simulink model "case3"  (Simulink 5.0)
settings: Solver=ode15s  SolverMode=SingleTasking  StartTime=0.0  StopTime=2  RelTol=1e-4  AbsTol=1e-3
InitFcn:
  | powericon('psbinitsys',bdroot);
StopFcn:
  | set_param(gcs,'Dirty','off')
undefined symbols (not defined in the file): A11, A12, A13, A14, A15, A16, A21, A22, A23, A24, A25, A26, A31, A32, A33, A34, A35, A36, A41, A42, A43, A44, A45, A46, A51, A52, A53, A54, A55, A56, A61, A62, A63, A64, A65, A66, A67, A81, A82, A92, g1, g2, g4, g9, gref, Le, po, Re, u01, u02, Wr
libraries: powerlib2 x14
settings Model: RequirementInfo=9  Creator=patrice  LastModifiedBy=pavel  ExtModeTrigMode=oneshot  ExtModeArmWhenConnect=off  InitialState=xinit  SaveTime=off  SaveOutput=off  FinalStateName=xinit  LimitDataPoints=off  IntegerOverflowMsg=none  BlockReductionOpt=off  BooleanDataType=off  RTWTemplateMakefile=grt_unix.tmf

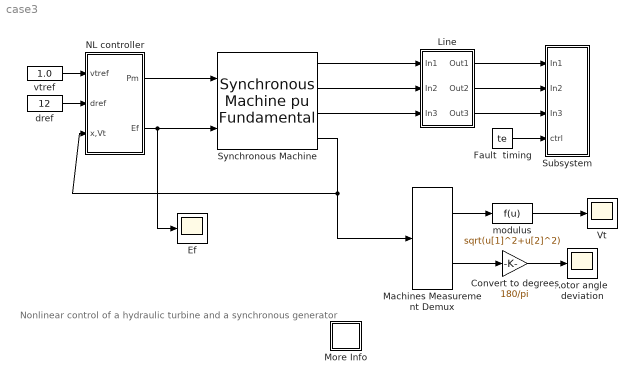
== system case3 ==
  note: Nonlinear control of a hydraulic turbine
      | and a synchronous generator
  Convert to degrees : Gain  Gain=180/pi  SaturateOnIntegerOverflow=on
  Ef : Scope
      settings: TickLabels=on  YMin=-12.5  YMax=12.5  DataFormat=Array
  Fault  timing : FromWorkspace  VariableName=te  SampleTime=0  mask( Fault timing){t=[0,0.1,0.2,0.4], e=[1,0,1,1]}
      mask prompts: t "transition steps:"; e "states (0/1):"
      mask help: steps
      mask init:
      | te=[t,t(2:length(t))-1e-8,t(length(t))+1e-8;e,e]';[y,i]=sort(te(:,1));te=[te(i,1),te(i,2)];
      mask Display: plot(te(:,1),te(:,2))
  Line : Subsystem
  Machines Measurement Demux : powerlib2/Machines/Machines Measurement Demux  machType=Synchronous  ssm1=on  ssm2=on  ssm3=on  ssm4=on  ssm5=on  ssm6=on  sm1=off  sm2=off  sm3=off  sm4=off  sm5=off  sm6=on  sm7=on  sm8=off  sm9=off  sm10=off  sm11=off  sm115=off  sm12=off  sm13=off  sm14=off  asm1=on  asm2=on  asm3=on  asm4=on  asm5=on  asm6=on  asm7=on  asm8=on  asm9=on  asm10=on  asm11=on  pmsm1=on  pmsm2=on  pmsm3=on  pmsm4=on  pmsm5=on  pmsm6=on  lastType=1
  More Info : Subsystem
      mask Display: disp('?')
  NL controller : Subsystem  mask(Non-linear speed and excitation controller){K=1, etat=1, mac=psbregulator/Synchronous Machine, delta=12, sm=[ 10/3  0.07 ], gate=[  0.01  0.97518  -0.1  0.1 ], Tw=2.67}
      mask prompts: K "Bus voltage (p.u.):"; etat "Controller state (0=off,1=on):"; mac "Associated machine name:"; delta "Desired load angle (deg):"; sm "Servo-motor [ Ka()  Ta(sec) ]:"; gate "Gate opening limits [ gmin,gmax(pu)    vgmin,vgmax(pu/s) ]:"; Tw "Water time constant Tw(sec):"
      mask init:
      | a=pi/2;[A11,A12,A13,A14,A15,A16,A21,A22,A23,A24,A25,A26,A31,A32,A33,A34,A35,A36,A41,A42,A43,A44,A45,A46,A51,A52,A53,A54,A55,A56,A61,A62,A63,A64,A65,A66,A67,A81,A82,A92,g1,g2,g4,g9,u01,u02,Re,Le,Wr,gref,po]=psbregulset(K,mac,delta);Ka=sm(1);Ta=sm(2);gmin=gate(1);gmax=gate(2);vgmin=gate(3);vgmax=gate(4);go=po*(gmax-gmin);
  Rotor angle  deviation : Scope
      settings: TickLabels=on  TimeRange=2  YMin=10.5  YMax=13.5  DataFormat=Array  Decimation=10
  Subsystem : Subsystem
  Synchronous Machine : powerlib2/Machines/Synchronous Machine pu Fundamental  Tag=PoWeRsYsTeMbLoCk  rotorType=Salient-pole  x1="[ 202E6  13800   60 ]"  x2="[ 0.003   0.19837   0.91763   0.21763 ]"  x3="[ 6.3581E-04   0.16537 ]"  x4b=[]  x4="[ 4.6454E-03  3.9203E-02  6.8430E-03  1.4544E-02 ]"  x5="[ 3.195  0  32 ]"  x6=[0 12 0.30512 0.30512 0.30512 105.77 -14.23 -134.23 0.970463]  x7=off  x8=[ ]  PSBOutputType=1110  iounits=0  LoadFlowParameters=[1,0,0,0,0]
  Vt : Scope
      settings: TickLabels=on  TimeRange=2  YMin=5.55112e-017  YMax=1.6  SaveName=ScopeData2  DataFormat=Array
  dref : Constant  Value=12
  modulus : Fcn  Expr=sqrt(u[1]^2+u[2]^2)
  vtref : Constant  Value=1.0
  wires:
  Synchronous Machine/3 -> Line/3(In3)
  Synchronous Machine/1 -> Line/1(In1)
  Synchronous Machine/2 -> Line/2(In2)
  Synchronous Machine/4 -> NL controller/3(x,Vt), Machines Measurement Demux/1
  dref/1 -> NL controller/2(dref)
  NL controller/2(Ef) -> Synchronous Machine/2, Ef/1
  vtref/1 -> NL controller/1(vtref)
  NL controller/1(Pm) -> Synchronous Machine/1
  Line/1(Out1) -> Subsystem/1(In1)
  Line/2(Out2) -> Subsystem/2(In2)
  Line/3(Out3) -> Subsystem/3(In3)
  Fault  timing/1 -> Subsystem/4(ctrl)
  Machines Measurement Demux/2 -> Convert to degrees/1
  Machines Measurement Demux/1 -> modulus/1
  modulus/1 -> Vt/1
  Convert to degrees/1 -> Rotor angle  deviation/1

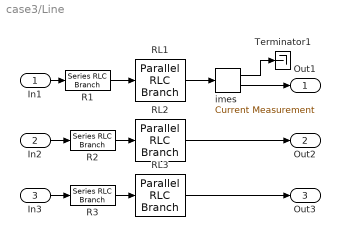
== system case3/Line ==
  In1 : Inport
  In2 : Inport  Port=2
  In3 : Inport  Port=3
  R1 : powerlib2/Elements/Series RLC Branch  Tag=PoWeRsYsTeMbLoCk  a=5.6566e-2  b=0  c=inf  mesure=None  PSBOutputType=1
  R2 : powerlib2/Elements/Series RLC Branch  Tag=PoWeRsYsTeMbLoCk  a=5.6566e-2  b=0  c=inf  mesure=None  PSBOutputType=1
  R3 : powerlib2/Elements/Series RLC Branch  Tag=PoWeRsYsTeMbLoCk  a=5.6566e-2  b=0  c=inf  mesure=None  PSBOutputType=1
  RL1 : powerlib2/Elements/Parallel RLC Branch  Tag=PoWeRsYsTeMbLoCk  a=25  b=6.5668e-4  c=0  mesure=None  PSBOutputType=1
  RL2 : powerlib2/Elements/Parallel RLC Branch  Tag=PoWeRsYsTeMbLoCk  a=25  b=6.5668e-4  c=0  mesure=None  PSBOutputType=1
  RL3 : powerlib2/Elements/Parallel RLC Branch  Tag=PoWeRsYsTeMbLoCk  a=25  b=6.5668e-4  c=0  mesure=None  PSBOutputType=1
  Terminator1 : Terminator
  imes : powerlib2/Measurements/Current Measurement  Tag=PoWeRsYsTeMmEaSuReMeNt  PhasorSimulation=off  OutputType=Magnitude  PSBOutputType=01  PSBequivalent=1
  Out1 : Outport  InitialOutput=0
  Out2 : Outport  Port=2  InitialOutput=0
  Out3 : Outport  Port=3  InitialOutput=0
  wires:
  imes/1 -> Terminator1/1
  RL3/1 -> Out3/1
  RL2/1 -> Out2/1
  In1/1 -> R1/1
  In2/1 -> R2/1
  In3/1 -> R3/1
  RL1/1 -> imes/1
  imes/2 -> Out1/1
  R1/1 -> RL1/1
  R2/1 -> RL2/1
  R3/1 -> RL3/1

== system case3/More Info ==
  note: Aime Francis Okou and Louis-A. Dessaint (École de technologie superieure, Montréal)
  note: 3
  note: Case study: Synchronous Machine and Regulator
  note: Circuit Description
  note: Demonstration
  note: This case study investigates the application of a multi-input multi-output nonlinear controller to a system consisting of a hydraulic
      | turbine and a synchronous generator connected to an infinite bus. The complete system is modeled using SimPowerSystems
      | and Simulink blocks. The controller is based on a feedback linearization scheme. Its main goal is to control the rotor angle as well as
      | the terminal voltage, to improve the stability properties, and to obtain good dynamic response.
      |
      | The performance of the nonlinear controller is tested on the nonlinear turbine-generator system. The controller and turbine are
      | simulated using Simulink blocks while the generator is represented by the Synchronous Machine block from the powerlib library.
      | A three-phase short-circuit is simulated on the load busbar and the fault is cleared after 100 ms.
  note: 1
  note: 2
  note: Start the simulation. Observe the field voltage Ef, power angle delta, and terminal voltage Vt.
  note: References
  note: You can observe how the stabilization of Vt is obtained in less than 0.25 seconds with this controller.
      | The load angle takes longer to stabilize, because the time constant of the mechanical part of the system
      | is much larger than the electrical time constants.
  note: If you want to compare results with classical regulators, replace the nonlinear controller with the same
      | excitation system and Hydraulic Turbine and Governor block used in the psbturbine demo. You will notice
      | that the system takes longer to stabilize than in this case study.
  note: Akhrif O., A.F. Okou, L.A. Dessaint, and R. Champagne, "Application of a Multivariable Feedback Linearization
      | Scheme for Rotor Angle Stability and Voltage Regulation of Power Systems", IEEE Transactions on Power Systems,
      | vol. 14, no. 2, May 1999, pp. 620-628.

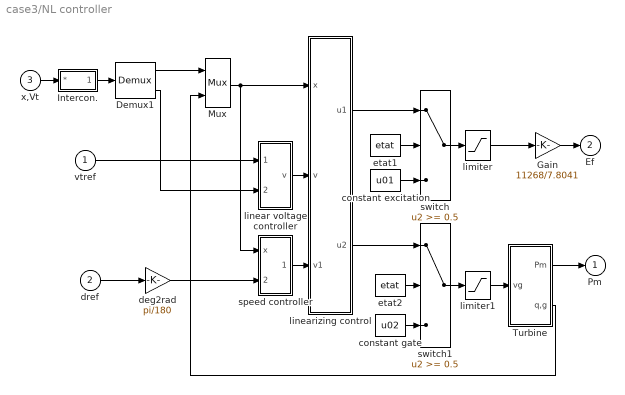
== system case3/NL controller ==
  vtref : Inport
  dref : Inport  Port=2
  x,Vt : Inport  Port=3
  Demux1 : Demux  Outputs=[7,1]
  Gain : Gain  Gain=11268/7.8041  SaturateOnIntegerOverflow=on
  Intercon. : Subsystem
  Mux : Mux  Inputs=[7,2]
  Turbine : Subsystem
  constant excitation : Constant  Value=u01
  constant gate : Constant  Value=u02
  deg2rad : Gain  Gain=pi/180  SaturateOnIntegerOverflow=on
  etat1 : Constant  Value=etat
  etat2 : Constant  Value=etat
  limiter : Saturate  UpperLimit=11.5*7.804/11268  LowerLimit=-11.5*7.804/11268  ZeroCross=off
  limiter1 : Saturate  UpperLimit=1  LowerLimit=-1  ZeroCross=off
  linear voltage controller : Subsystem
  linearizing control : Subsystem
  speed controller : Subsystem
  switch : Switch  Threshold=0.5  ZeroCross=off  InputSameDT=on
  switch1 : Switch  Threshold=0.5  ZeroCross=off  InputSameDT=on
  Pm : Outport  InitialOutput=0
  Ef : Outport  Port=2  InitialOutput=0
  wires:
  vtref/1 -> linear voltage controller/1(vtref)
  deg2rad/1 -> speed controller/2(dref)
  Gain/1 -> Ef/1
  Turbine/1(Pm) -> Pm/1
  constant gate/1 -> switch1/3
  etat2/1 -> switch1/2
  linearizing control/2(u2) -> switch1/1
  constant excitation/1 -> switch/3
  etat1/1 -> switch/2
  linearizing control/1(u1) -> switch/1
  switch1/1 -> limiter1/1
  limiter1/1 -> Turbine/1(vg)
  limiter/1 -> Gain/1
  switch/1 -> limiter/1
  linear voltage controller/1(v) -> linearizing control/2(v)
  speed controller/1(v1) -> linearizing control/3(v1)
  x,Vt/1 -> Intercon./1(*)
  Demux1/2 -> linear voltage controller/2(vt)
  Demux1/1 -> Mux/1
  Turbine/2(q,g) -> Mux/2
  dref/1 -> deg2rad/1
  Mux/1 -> linearizing control/1(x), speed controller/1(x)
  Intercon./1(" x,vt ") -> Demux1/1

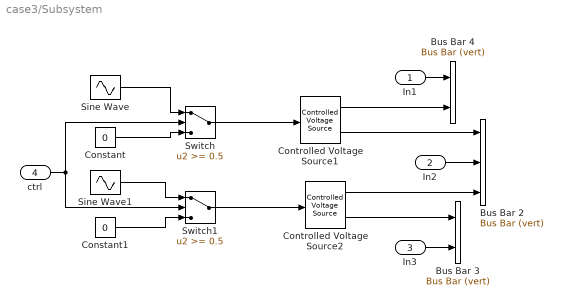
== system case3/Subsystem ==
  In1 : Inport
  In2 : Inport  Port=2
  In3 : Inport  Port=3
  ctrl : Inport  Port=4
  Bus Bar 2 : powerlib2/Connectors/Bus Bar (vert)  entrees=3  sorties=0  PSBOutputType=11111111111111111111111111111111111111111111111111111111111111111111111111111111111111111
  Bus Bar 3 : powerlib2/Connectors/Bus Bar (vert)  entrees=2  sorties=0  PSBOutputType=11111111111111111111111111111111111111111111111111111111111111111111111111111111111111111
  Bus Bar 4 : powerlib2/Connectors/Bus Bar (vert)  entrees=2  sorties=0  PSBOutputType=11111111111111111111111111111111111111111111111111111111111111111111111111111111111111111
  Constant : Constant  Value=0
  Constant1 : Constant  Value=0
  Controlled Voltage Source1 : powerlib2/Electrical Sources/Controlled Voltage Source  Tag=PoWeRsYsTeMbLoCk  initsrc=on  srctyp=AC  iv=13800*sqrt(2)*sin(60*2*pi+120*pi/180)  iph=0  ifreq=0  mesure=None  PSBOutputType=11
  Controlled Voltage Source2 : powerlib2/Electrical Sources/Controlled Voltage Source  Tag=PoWeRsYsTeMbLoCk  initsrc=on  srctyp=AC  iv=13800*sqrt(2)*sin(60*2*pi+0)  iph=0  ifreq=0  mesure=None  PSBOutputType=11
  Sine Wave : Sin  Amplitude=13800*sqrt(2)  Frequency=60*2*pi  Phase=120*pi/180  SampleTime=0
  Sine Wave1 : Sin  Amplitude=13800*sqrt(2)  Frequency=60*2*pi  SampleTime=0
  Switch : Switch  Threshold=0.5  ZeroCross=off  InputSameDT=on
  Switch1 : Switch  Threshold=0.5  ZeroCross=off  InputSameDT=on
  wires:
  Controlled Voltage Source2/2 -> Bus Bar 3/1
  Controlled Voltage Source2/1 -> Bus Bar 2/3
  Sine Wave1/1 -> Switch1/1
  Constant1/1 -> Switch1/3
  Switch1/1 -> Controlled Voltage Source2/1
  In3/1 -> Bus Bar 3/2
  Controlled Voltage Source1/2 -> Bus Bar 2/1
  Controlled Voltage Source1/1 -> Bus Bar 4/2
  Switch/1 -> Controlled Voltage Source1/1
  Constant/1 -> Switch/3
  Sine Wave/1 -> Switch/1
  ctrl/1 -> Switch1/2, Switch/2
  In1/1 -> Bus Bar 4/1
  In2/1 -> Bus Bar 2/2

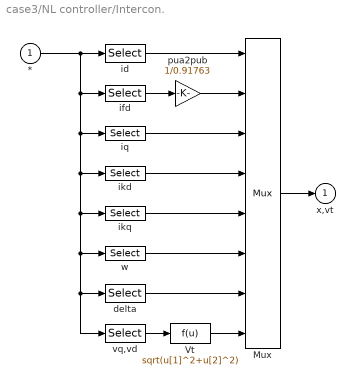
== system case3/NL controller/Intercon. ==
  * : Inport
  Mux : Mux  Inputs=8
  Vt : Fcn  Expr=sqrt(u[1]^2+u[2]^2)
  delta : Selector  Elements=14  InputPortWidth=22
  id : Selector  Elements=5  InputPortWidth=22
  ifd : Selector  Elements=6  InputPortWidth=22
  ikd : Selector  Elements=9  InputPortWidth=22
  ikq : Selector  Elements=7  InputPortWidth=22
  iq : Selector  Elements=4  InputPortWidth=22
  pua2pub : Gain  Gain=1/0.91763  SaturateOnIntegerOverflow=on
  vq,vd : Selector  Elements=[ 12:13 ]  InputPortWidth=22
  w : Selector  Elements=15  InputPortWidth=22
  " x,vt " : Outport  InitialOutput=0
  wires:
  w/1 -> Mux/6
  ikq/1 -> Mux/5
  ikd/1 -> Mux/4
  id/1 -> Mux/1
  iq/1 -> Mux/3
  Mux/1 -> " x,vt "/1
  vq,vd/1 -> Vt/1
  */1 -> id/1, ifd/1, iq/1, ikd/1, ikq/1, w/1, vq,vd/1, delta/1
  Vt/1 -> Mux/8
  ifd/1 -> pua2pub/1
  pua2pub/1 -> Mux/2
  delta/1 -> Mux/7

== system case3/NL controller/Turbine ==
  vg : Inport
  Mux : Mux  Inputs=2
  servo-motor : Subsystem
      mask Display: disp('servo-\nmotor')
  turbine : Subsystem
      mask Display: disp('hydraulic\nturbine')
  Pm : Outport  InitialOutput=0
  q,g : Outport  Port=2  InitialOutput=0
  wires:
  servo-motor/1(gate opening) -> Mux/2, turbine/1(gate opening)
  turbine/2(q) -> Mux/1
  turbine/1(Pm) -> Pm/1
  vg/1 -> servo-motor/1(regulator's output)
  Mux/1 -> q,g/1

== system case3/NL controller/linear voltage controller ==
  vtref : Inport
  vt : Inport  Port=2
  Gain : Gain  Gain=-7  SaturateOnIntegerOverflow=on
  Sum : Sum  Inputs=-+  SaturateOnIntegerOverflow=on  InputSameDT=on
  v : Outport  InitialOutput=0
  wires:
  Sum/1 -> Gain/1
  vtref/1 -> Sum/1
  Gain/1 -> v/1
  vt/1 -> Sum/2

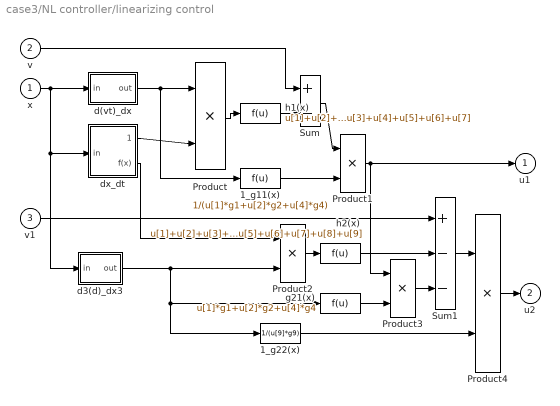
== system case3/NL controller/linearizing control ==
  x : Inport
  v : Inport  Port=2
  v1 : Inport  Port=3
  1_g11(x) : Fcn  Expr=1/(u[1]*g1+u[2]*g2+u[4]*g4)
  1_g22(x) : Fcn  Expr=1/(u[9]*g9)
  Product{,1..4} (5 alike) : Product  SaturateOnIntegerOverflow=on  InputSameDT=on
  Sum : Sum  Inputs=+-  SaturateOnIntegerOverflow=on  InputSameDT=on
  Sum1 : Sum  Inputs=+--  SaturateOnIntegerOverflow=on  InputSameDT=on
  d(vt)_dx : Subsystem
  d3(d)_dx3 : Subsystem
  dx_dt : Subsystem
  g21(x) : Fcn  Expr=u[1]*g1+u[2]*g2+u[4]*g4
  h1(x) : Fcn  Expr=u[1]+u[2]+u[3]+u[4]+u[5]+u[6]+u[7]
  h2(x) : Fcn  Expr=u[1]+u[2]+u[3]+u[4]+u[5]+u[6]+u[7]+u[8]+u[9]
  u1 : Outport  InitialOutput=0
  u2 : Outport  Port=2  InitialOutput=0
  wires:
  d3(d)_dx3/1(out) -> Product2/2, 1_g22(x)/1, g21(x)/1
  dx_dt/2(f(x)) -> Product2/1
  Product2/1 -> h2(x)/1
  h2(x)/1 -> Sum1/2
  g21(x)/1 -> Product3/2
  Product3/1 -> Sum1/3
  Sum1/1 -> Product4/1
  1_g22(x)/1 -> Product4/2
  Product4/1 -> u2/1
  v1/1 -> Sum1/1
  dx_dt/1(f(xms)) -> Product/2
  x/1 -> d(vt)_dx/1(in), d3(d)_dx3/1(in), dx_dt/1(in)
  Product1/1 -> u1/1, Product3/1
  Sum/1 -> Product1/1
  1_g11(x)/1 -> Product1/2
  d(vt)_dx/1(out) -> 1_g11(x)/1, Product/1
  h1(x)/1 -> Sum/2
  Product/1 -> h1(x)/1
  v/1 -> Sum/1

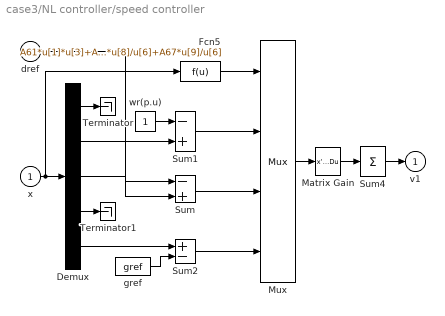
== system case3/NL controller/speed controller ==
  x : Inport
  dref : Inport  Port=2
  Demux : Demux  Outputs=[ 5,1,1,1,1]
  Fcn5 : Fcn  Expr=A61*u[1]*u[3]+A62*u[2]*u[3]+A63*u[3]*u[4]+A64*u[1]*u[5]+A65*u[6]+A66*u[8]/u[6]+A67*u[9]/u[6]
  Matrix Gain : StateSpace  A=[]  B=[]  C=[]  D=K  mask(Matrix Gain){@1=[ -Wr*11.00, -Wr*46.6345, -36.6345, 553.6311*80 ]}
      mask prompts: @1 "Gain matrix:"
      mask help: Matrix Gain.
      mask init:
      | K=@1;
      mask Help: Multiplies input vector by entered matrix to produce output vector (y=Au).
      mask Display: disp('K')
  Mux : Mux
  Sum : Sum  Inputs=-+  SaturateOnIntegerOverflow=on  InputSameDT=on
  Sum1 : Sum  Inputs=-+  SaturateOnIntegerOverflow=on  InputSameDT=on
  Sum2 : Sum  Inputs=+-  SaturateOnIntegerOverflow=on  InputSameDT=on
  Sum4 : Sum  Inputs=+  SaturateOnIntegerOverflow=on  InputSameDT=on
  Terminator : Terminator
  Terminator1 : Terminator
  gref : Constant  Value=gref
  wr(p.u) : Constant
  v1 : Outport  InitialOutput=0
  wires:
  dref/1 -> Sum/1
  wr(p.u)/1 -> Sum1/1
  Sum1/1 -> Mux/2
  Sum2/1 -> Mux/4
  Fcn5/1 -> Mux/1
  gref/1 -> Sum2/2
  Sum/1 -> Mux/3
  Mux/1 -> Matrix Gain/1
  Matrix Gain/1 -> Sum4/1
  Sum4/1 -> v1/1
  Demux/4 -> Terminator1/1
  Demux/1 -> Terminator/1
  Demux/5 -> Sum2/1
  Demux/3 -> Sum/2
  Demux/2 -> Sum1/2
  x/1 -> Demux/1, Fcn5/1

== system case3/NL controller/Turbine/servo-motor ==
  regulator's output : Inport
  Integrator1 : Integrator  InitialCondition=go  ZeroCross=off
  Sum4 : Sum  Inputs=+-  SaturateOnIntegerOverflow=on  InputSameDT=on
  position limit : Saturate  UpperLimit=gmax  LowerLimit=gmin  ZeroCross=off
  servo motor : TransferFcn  Numerator=[Ka]  Denominator="[ Ta  1]"
  speed limit : Saturate  UpperLimit=vgmax  LowerLimit=vgmin  ZeroCross=off
  gate opening : Outport  InitialOutput=0
  wires:
  position limit/1 -> Sum4/2, gate opening/1
  Integrator1/1 -> position limit/1
  speed limit/1 -> Integrator1/1
  servo motor/1 -> speed limit/1
  Sum4/1 -> servo motor/1
  regulator's output/1 -> Sum4/1

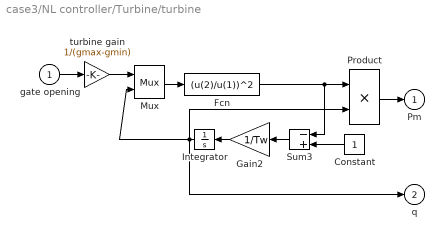
== system case3/NL controller/Turbine/turbine ==
  gate opening : Inport
  Constant : Constant  Orientation=left
  Fcn : Fcn  Expr=(u(2)/u(1))^2
  Gain2 : Gain  Orientation=left  Gain=1/Tw  SaturateOnIntegerOverflow=on
  Integrator : Integrator  Orientation=left  InitialCondition=po  ZeroCross=off
  Mux : Mux  Inputs=2
  Product : Product  SaturateOnIntegerOverflow=on  InputSameDT=on
  Sum3 : Sum  Orientation=left  Inputs=-+  SaturateOnIntegerOverflow=on  InputSameDT=on
  turbine gain : Gain  Gain=1/(gmax-gmin)  SaturateOnIntegerOverflow=on
  Pm : Outport  InitialOutput=0
  q : Outport  Port=2  InitialOutput=0
  wires:
  Integrator/1 -> q/1, Product/2, Mux/2
  Mux/1 -> Fcn/1
  Constant/1 -> Sum3/2
  Product/1 -> Pm/1
  Sum3/1 -> Gain2/1
  Gain2/1 -> Integrator/1
  turbine gain/1 -> Mux/1
  Fcn/1 -> Sum3/1, Product/1
  gate opening/1 -> turbine gain/1

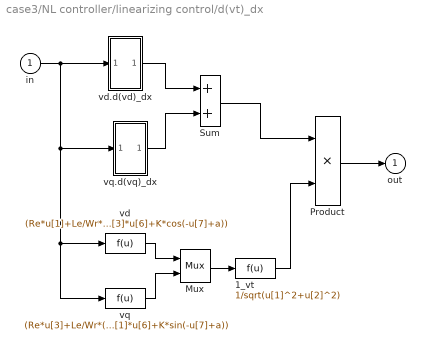
== system case3/NL controller/linearizing control/d(vt)_dx ==
  in : Inport
  1_vt : Fcn  Expr=1/sqrt(u[1]^2+u[2]^2)
  Mux : Mux  Inputs=2
  Product : Product  SaturateOnIntegerOverflow=on  InputSameDT=on
  Sum : Sum  SaturateOnIntegerOverflow=on  InputSameDT=on
  vd : Fcn  Expr=(Re*u[1]+Le/Wr*(A11*u[1]+A12*u[2]+A13*u[3]*u[6]+A14*u[4]+A15*u[5]*u[6]+A16*cos(-u[7]+a))-Le*u[3]*u[6]+K*cos(-u[7]+a))
  vd.d(vd)_dx : Subsystem
  vq : Fcn  Expr=(Re*u[3]+Le/Wr*(A31*u[1]*u[6]+A32*u[2]*u[6]+A33*u[3]+A34*u[4]*u[6]+A35*u[5]+A36*sin(-u[7]+a))+Le*u[1]*u[6]+K*sin(-u[7]+a))
  vq.d(vq)_dx : Subsystem
  out : Outport  InitialOutput=0
  wires:
  vd/1 -> Mux/1
  vq/1 -> Mux/2
  Mux/1 -> 1_vt/1
  in/1 -> vd/1, vq/1, vq.d(vq)_dx/1(in_1), vd.d(vd)_dx/1(in_1)
  vd.d(vd)_dx/1(out_1) -> Sum/1
  vq.d(vq)_dx/1(out_1) -> Sum/2
  1_vt/1 -> Product/2
  Sum/1 -> Product/1
  Product/1 -> out/1

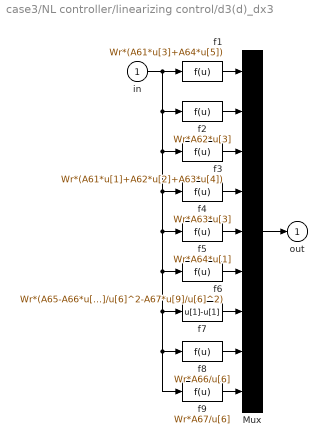
== system case3/NL controller/linearizing control/d3(d)_dx3 ==
  in : Inport
  Mux : Mux  Inputs=9
  f1 : Fcn  Expr=Wr*(A61*u[3]+A64*u[5])
  f2 : Fcn  Expr=Wr*A62*u[3]
  f3 : Fcn  Expr=Wr*(A61*u[1]+A62*u[2]+A63*u[4])
  f4 : Fcn  Expr=Wr*A63*u[3]
  f5 : Fcn  Expr=Wr*A64*u[1]
  f6 : Fcn  Expr=Wr*(A65-A66*u[8]/u[6]^2-A67*u[9]/u[6]^2)
  f7 : Fcn  Expr=u[1]-u[1]
  f8 : Fcn  Expr=Wr*A66/u[6]
  f9 : Fcn  Expr=Wr*A67/u[6]
  out : Outport  InitialOutput=0
  wires:
  Mux/1 -> out/1
  f7/1 -> Mux/7
  f6/1 -> Mux/6
  f5/1 -> Mux/5
  f4/1 -> Mux/4
  f3/1 -> Mux/3
  f2/1 -> Mux/2
  f1/1 -> Mux/1
  f8/1 -> Mux/8
  f9/1 -> Mux/9
  in/1 -> f2/1, f3/1, f4/1, f5/1, f6/1, f9/1, f8/1, f7/1, f1/1

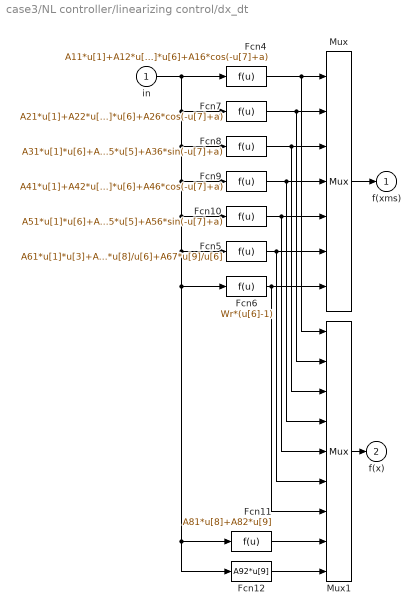
== system case3/NL controller/linearizing control/dx_dt ==
  in : Inport
  Fcn10 : Fcn  Expr=A51*u[1]*u[6]+A52*u[2]*u[6]+A53*u[3]+A54*u[4]*u[6]+A55*u[5]+A56*sin(-u[7]+a)
  Fcn11 : Fcn  Expr=A81*u[8]+A82*u[9]
  Fcn12 : Fcn  Expr=A92*u[9]
  Fcn4 : Fcn  Expr=A11*u[1]+A12*u[2]+A13*u[3]*u[6]+A14*u[4]+A15*u[5]*u[6]+A16*cos(-u[7]+a)
  Fcn5 : Fcn  Expr=A61*u[1]*u[3]+A62*u[2]*u[3]+A63*u[3]*u[4]+A64*u[1]*u[5]+A65*u[6]+A66*u[8]/u[6]+A67*u[9]/u[6]
  Fcn6 : Fcn  Expr=Wr*(u[6]-1)
  Fcn7 : Fcn  Expr=A21*u[1]+A22*u[2]+A23*u[3]*u[6]+A24*u[4]+A25*u[5]*u[6]+A26*cos(-u[7]+a)
  Fcn8 : Fcn  Expr=A31*u[1]*u[6]+A32*u[2]*u[6]+A33*u[3]+A34*u[4]*u[6]+A35*u[5]+A36*sin(-u[7]+a)
  Fcn9 : Fcn  Expr=A41*u[1]+A42*u[2]+A43*u[3]*u[6]+A44*u[4]+A45*u[5]*u[6]+A46*cos(-u[7]+a)
  Mux : Mux  Inputs=7
  Mux1 : Mux  Inputs=9
  f(xms) : Outport  InitialOutput=0
  f(x) : Outport  Port=2  InitialOutput=0
  wires:
  Mux/1 -> f(xms)/1
  Mux1/1 -> f(x)/1
  Fcn6/1 -> Mux/7, Mux1/7
  Fcn5/1 -> Mux/6, Mux1/6
  in/1 -> Fcn7/1, Fcn8/1, Fcn9/1, Fcn10/1, Fcn5/1, Fcn12/1, Fcn11/1, Fcn6/1, Fcn4/1
  Fcn12/1 -> Mux1/9
  Fcn11/1 -> Mux1/8
  Fcn10/1 -> Mux1/5, Mux/5
  Fcn9/1 -> Mux1/4, Mux/4
  Fcn8/1 -> Mux1/3, Mux/3
  Fcn7/1 -> Mux1/2, Mux/2
  Fcn4/1 -> Mux1/1, Mux/1

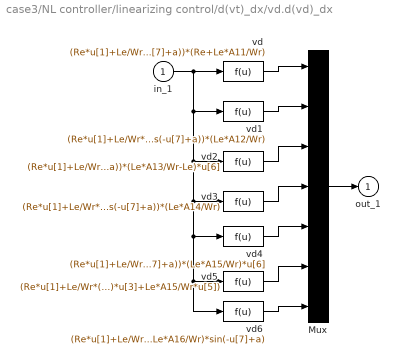
== system case3/NL controller/linearizing control/d(vt)_dx/vd.d(vd)_dx ==
  in_1 : Inport
  Mux : Mux  Inputs=7
  vd : Fcn  Expr=(Re*u[1]+Le/Wr*(A11*u[1]+A12*u[2]+A13*u[3]*u[6]+A14*u[4]+A15*u[5]*u[6]+A16*cos(-u[7]+a))-Le*u[3]*u[6]+K*cos(-u[7]+a))*(Re+Le*A11/Wr)
  vd1 : Fcn  Expr=(Re*u[1]+Le/Wr*(A11*u[1]+A12*u[2]+A13*u[3]*u[6]+A14*u[4]+A15*u[5]*u[6]+A16*cos(-u[7]+a))-Le*u[3]*u[6]+K*cos(-u[7]+a))*(Le*A12/Wr)
  vd2 : Fcn  Expr=(Re*u[1]+Le/Wr*(A11*u[1]+A12*u[2]+A13*u[3]*u[6]+A14*u[4]+A15*u[5]*u[6]+A16*cos(-u[7]+a))-Le*u[3]*u[6]+K*cos(-u[7]+a))*(Le*A13/Wr-Le)*u[6]
  vd3 : Fcn  Expr=(Re*u[1]+Le/Wr*(A11*u[1]+A12*u[2]+A13*u[3]*u[6]+A14*u[4]+A15*u[5]*u[6]+A16*cos(-u[7]+a))-Le*u[3]*u[6]+K*cos(-u[7]+a))*(Le*A14/Wr)
  vd4 : Fcn  Expr=(Re*u[1]+Le/Wr*(A11*u[1]+A12*u[2]+A13*u[3]*u[6]+A14*u[4]+A15*u[5]*u[6]+A16*cos(-u[7]+a))-Le*u[3]*u[6]+K*cos(-u[7]+a))*(Le*A15/Wr)*u[6]
  vd5 : Fcn  Expr=(Re*u[1]+Le/Wr*(A11*u[1]+A12*u[2]+A13*u[3]*u[6]+A14*u[4]+A15*u[5]*u[6]+A16*cos(-u[7]+a))-Le*u[3]*u[6]+K*cos(-u[7]+a))*((Le*A13/Wr-Le)*u[3]+Le*A15/Wr*u[5])
  vd6 : Fcn  Expr=(Re*u[1]+Le/Wr*(A11*u[1]+A12*u[2]+A13*u[3]*u[6]+A14*u[4]+A15*u[5]*u[6]+A16*cos(-u[7]+a))-Le*u[3]*u[6]+K*cos(-u[7]+a))*(K+Le*A16/Wr)*sin(-u[7]+a)
  out_1 : Outport  InitialOutput=0
  wires:
  Mux/1 -> out_1/1
  in_1/1 -> vd5/1, vd6/1, vd4/1, vd3/1, vd2/1, vd1/1, vd/1
  vd/1 -> Mux/1
  vd1/1 -> Mux/2
  vd2/1 -> Mux/3
  vd3/1 -> Mux/4
  vd4/1 -> Mux/5
  vd5/1 -> Mux/6
  vd6/1 -> Mux/7

== system case3/NL controller/linearizing control/d(vt)_dx/vq.d(vq)_dx ==
  in_1 : Inport
  Mux : Mux  Inputs=7
  vq : Fcn  Expr=(Re*u[3]+Le/Wr*(A31*u[1]*u[6]+A32*u[2]*u[6]+A33*u[3]+A34*u[4]*u[6]+A35*u[5]+A36*sin(-u[7]+a))+Le*u[1]*u[6]+K*sin(-u[7]+a))*(Le*A31/Wr+Le)*u[6]
  vq1 : Fcn  Expr=(Re*u[3]+Le/Wr*(A31*u[1]*u[6]+A32*u[2]*u[6]+A33*u[3]+A34*u[4]*u[6]+A35*u[5]+A36*sin(-u[7]+a))+Le*u[1]*u[6]+K*sin(-u[7]+a))*Le*A32/Wr*u[6]
  vq2 : Fcn  Expr=(Re*u[3]+Le/Wr*(A31*u[1]*u[6]+A32*u[2]*u[6]+A33*u[3]+A34*u[4]*u[6]+A35*u[5]+A36*sin(-u[7]+a))+Le*u[1]*u[6]+K*sin(-u[7]+a))*(Re+Le*A33/Wr)
  vq3 : Fcn  Expr=(Re*u[3]+Le/Wr*(A31*u[1]*u[6]+A32*u[2]*u[6]+A33*u[3]+A34*u[4]*u[6]+A35*u[5]+A16*sin(-u[7]+a))+Le*u[1]*u[6]+K*sin(-u[7]+a))*(Le*A34/Wr)*u[6]
  vq4 : Fcn  Expr=(Re*u[3]+Le/Wr*(A31*u[1]*u[6]+A32*u[2]*u[6]+A33*u[3]+A34*u[4]*u[6]+A35*u[5]+A36*sin(-u[7]+a))+Le*u[1]*u[6]+K*sin(-u[7]+a))*(Le*A35/Wr)
  vq5 : Fcn  Expr=(Re*u[3]+Le/Wr*(A31*u[1]*u[6]+A32*u[2]*u[6]+A33*u[3]+A34*u[4]*u[6]+A35*u[5]+A36*sin(-u[7]+a))+Le*u[1]*u[6]+K*sin(-u[7]+a))*((Le+Le*A31/Wr)*u[1]+Le*A32/Wr*u[2]+Le*A34/Wr*u[4])
  vq6 : Fcn  Expr=(Re*u[3]+Le/Wr*(A31*u[1]*u[6]+A32*u[2]*u[6]+A33*u[3]+A34*u[4]*u[6]+A35*u[5]+A36*sin(-u[7]+a))+Le*u[1]*u[6]+K*sin(-u[7]+a))*(-cos(-u[7]+a)*(Le*A36/Wr+K))
  out_1 : Outport  InitialOutput=0
  wires:
  Mux/1 -> out_1/1
  in_1/1 -> vq5/1, vq6/1, vq4/1, vq3/1, vq2/1, vq1/1, vq/1
  vq/1 -> Mux/1
  vq1/1 -> Mux/2
  vq2/1 -> Mux/3
  vq3/1 -> Mux/4
  vq4/1 -> Mux/5
  vq5/1 -> Mux/6
  vq6/1 -> Mux/7
